simulink model "me132LabPartC"  (R2021a)
settings: Solver=VariableStepAuto  StartTime=0.0  StopTime=10.0  RelTol=1e-3
undefined symbols (not defined in the file or in its folder): c3
settings Model: Creator=kaiyu  LastModifiedBy=kaiyu

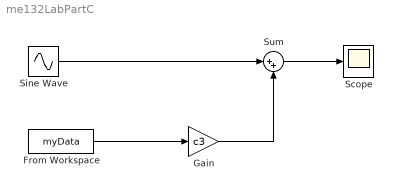
== system me132LabPartC ==
  From Workspace : FromWorkspace  VariableName=myData
  Gain : Gain  Gain=c3
  Scope : Scope
  Sine Wave : Sin  Amplitude=0.2  Frequency=10  SampleTime=0
  Sum : Sum  Inputs=|++
  wires:
  From Workspace/1 -> Gain/1
  Gain/1 -> Sum/2
  Sine Wave/1 -> Sum/1
  Sum/1 -> Scope/1
